simulink model "system_simulation"  (Simulink 8.9)
settings: Solver=ode4  StartTime=0.0  StopTime=300  FixedStep=0.01  RelTol=1e-3  EnableMultiTasking=on
values from neighbouring files (symbols this model uses):
  alpha_0 = 10*pi/180    (= 0.174532925199)    [para_initial.m]
  attitude_angle_0 = [5*pi/180;3*pi/180;-5*pi/180]    [para_initial.m]
  beta_0 = -10*pi/180    (= -0.174532925199)    [para_initial.m]
  omega_0 = 0.00075563    [para_initial.m]
  u_0 = [0;0;0;0;0;0;0;0]    [para_initial.m]
settings Model: Creator=Administrator  LastModifiedBy=yyywxk
settings DataIOCC: SignalLoggingSaveFormat=Dataset
settings DebuggingCC: SolverPrmCheckMsg=warning  MultiTaskDSMMsg=warning  MultiTaskCondExecSysMsg=none
settings GRTTargetCC: CombineOutputUpdateFcns=on  GRTInterface=off

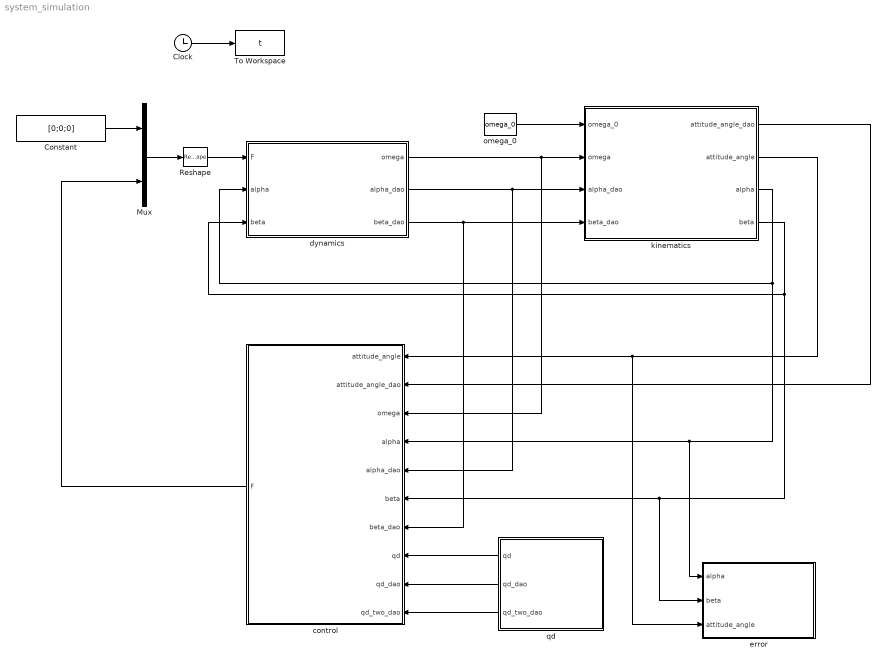
== system system_simulation ==
  Clock : Clock
  Constant : Constant  Value=[0;0;0]
  Mux : Mux  Inputs=2
  Reshape : Reshape
  To Workspace : ToWorkspace  VariableName=t  SampleTime=-1
  control : Subsystem
  dynamics : Subsystem
  error : Subsystem
  kinematics : Subsystem
  omega_0 : Constant  Value=omega_0
  qd : Subsystem
  wires:
  Clock/1 -> To Workspace/1
  dynamics/2(alpha_dao) -> control/5(alpha_dao), kinematics/3(alpha_dao)
  dynamics/1(omega) -> control/3(omega), kinematics/2(omega)
  omega_0/1 -> kinematics/1(omega_0)
  kinematics/3(alpha) -> dynamics/2(alpha), error/1(alpha), control/4(alpha)
  kinematics/2(attitude_angle) -> error/3(attitude_angle), control/1(attitude_angle)
  kinematics/1(attitude_angle_dao) -> control/2(attitude_angle_dao)
  Mux/1 -> Reshape/1
  Constant/1 -> Mux/1
  control/1(F) -> Mux/2
  Reshape/1 -> dynamics/1(F)
  dynamics/3(beta_dao) -> control/7(beta_dao), kinematics/4(beta_dao)
  qd/2(qd_dao) -> control/9(qd_dao)
  qd/1(qd) -> control/8(qd)
  qd/3(qd_two_dao) -> control/10(qd_two_dao)
  kinematics/4(beta) -> dynamics/3(beta), error/2(beta), control/6(beta)

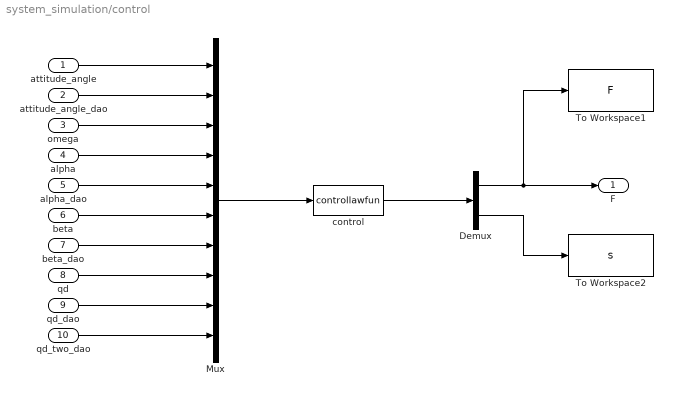
== system system_simulation/control ==
  attitude_angle : Inport
  attitude_angle_dao : Inport  Port=2
  omega : Inport  Port=3
  alpha : Inport  Port=4
  alpha_dao : Inport  Port=5
  beta : Inport  Port=6
  beta_dao : Inport  Port=7
  qd : Inport  Port=8
  qd_dao : Inport  Port=9
  qd_two_dao : Inport  Port=10
  Demux : Demux  Outputs=2
  Mux : Mux  Inputs=10
  To Workspace1 : ToWorkspace  VariableName=F  SampleTime=-1
  To Workspace2 : ToWorkspace  VariableName=s  SampleTime=-1
  control : MATLABFcn  MATLABFcn=controllawfun  OutputDimensions=10
  F : Outport
  wires:
  Mux/1 -> control/1
  attitude_angle/1 -> Mux/1
  attitude_angle_dao/1 -> Mux/2
  omega/1 -> Mux/3
  alpha/1 -> Mux/4
  alpha_dao/1 -> Mux/5
  qd/1 -> Mux/8
  qd_dao/1 -> Mux/9
  qd_two_dao/1 -> Mux/10
  control/1 -> Demux/1
  Demux/1 -> F/1, To Workspace1/1
  Demux/2 -> To Workspace2/1
  beta/1 -> Mux/6
  beta_dao/1 -> Mux/7

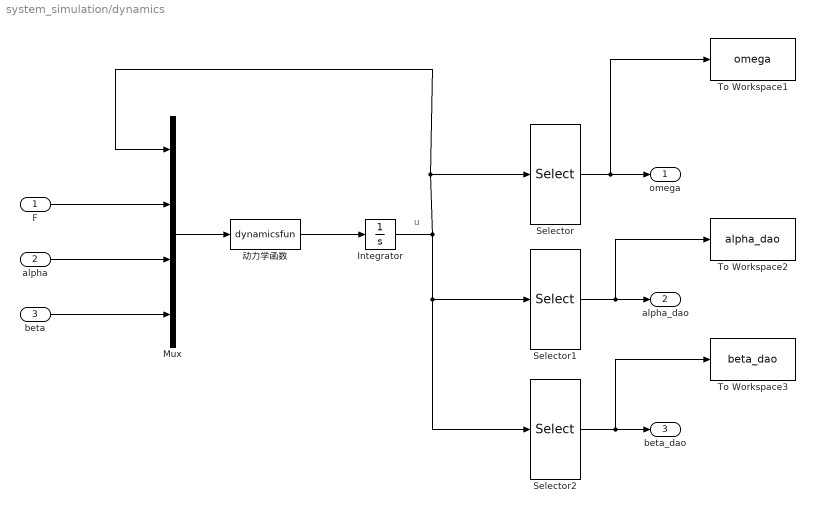
== system system_simulation/dynamics ==
  note: u
  F : Inport
  alpha : Inport  Port=2
  beta : Inport  Port=3
  Integrator : Integrator  InitialCondition=u_0
  Mux : Mux
  Selector : Selector  InputPortWidth=8  IndexOptions=Index vector (dialog)  Indices=[4 5 6]  OutputSizes=1
  Selector1 : Selector  InputPortWidth=8  IndexOptions=Index vector (dialog)  Indices=[7]  OutputSizes=1
  Selector2 : Selector  InputPortWidth=8  IndexOptions=Index vector (dialog)  Indices=[8]  OutputSizes=1
  To Workspace1 : ToWorkspace  VariableName=omega  SampleTime=-1
  To Workspace2 : ToWorkspace  VariableName=alpha_dao  SampleTime=-1
  To Workspace3 : ToWorkspace  VariableName=beta_dao  SampleTime=-1
  动力学函数 : MATLABFcn  MATLABFcn=dynamicsfun  OutputDimensions=8
  omega : Outport
  alpha_dao : Outport  Port=2
  beta_dao : Outport  Port=3
  wires:
  Mux/1 -> 动力学函数/1
  F/1 -> Mux/2
  alpha/1 -> Mux/3
  动力学函数/1 -> Integrator/1
  Integrator/1 -> Selector2/1, Selector1/1, Mux/1, Selector/1
  Selector/1 -> omega/1, To Workspace1/1
  Selector1/1 -> alpha_dao/1, To Workspace2/1
  Selector2/1 -> To Workspace3/1, beta_dao/1
  beta/1 -> Mux/4

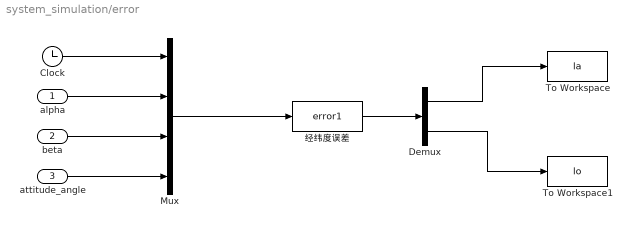
== system system_simulation/error ==
  alpha : Inport
  beta : Inport  Port=2
  attitude_angle : Inport  Port=3
  Clock : Clock
  Demux : Demux  Outputs=2
  Mux : Mux
  To Workspace : ToWorkspace  VariableName=la  SampleTime=-1
  To Workspace1 : ToWorkspace  VariableName=lo  SampleTime=-1
  经纬度误差 : MATLABFcn  MATLABFcn=error1  OutputDimensions=2
  wires:
  Clock/1 -> Mux/1
  Mux/1 -> 经纬度误差/1
  经纬度误差/1 -> Demux/1
  Demux/1 -> To Workspace/1
  Demux/2 -> To Workspace1/1
  alpha/1 -> Mux/2
  beta/1 -> Mux/3
  attitude_angle/1 -> Mux/4

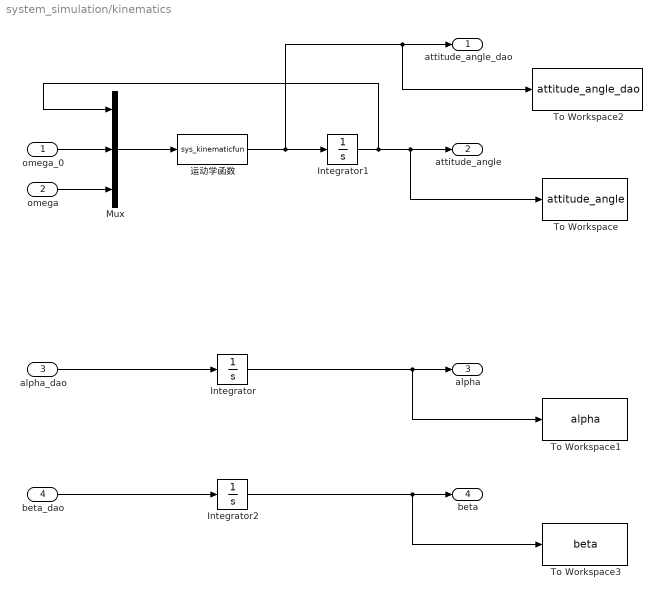
== system system_simulation/kinematics ==
  omega_0 : Inport
  omega : Inport  Port=2
  alpha_dao : Inport  Port=3
  beta_dao : Inport  Port=4
  Integrator : Integrator  InitialCondition=alpha_0
  Integrator1 : Integrator  InitialCondition=attitude_angle_0
  Integrator2 : Integrator  InitialCondition=beta_0
  Mux : Mux  Inputs=3
  To Workspace : ToWorkspace  VariableName=attitude_angle  SampleTime=-1
  To Workspace1 : ToWorkspace  VariableName=alpha  SampleTime=-1
  To Workspace2 : ToWorkspace  VariableName=attitude_angle_dao  SampleTime=-1
  To Workspace3 : ToWorkspace  VariableName=beta  SampleTime=-1
  运动学函数 : MATLABFcn  MATLABFcn=sys_kinematicfun  OutputDimensions=3
  attitude_angle_dao : Outport
  attitude_angle : Outport  Port=2
  alpha : Outport  Port=3
  beta : Outport  Port=4
  wires:
  Integrator/1 -> alpha/1, To Workspace1/1
  Integrator1/1 -> To Workspace/1, attitude_angle/1, Mux/1
  omega_0/1 -> Mux/2
  alpha_dao/1 -> Integrator/1
  omega/1 -> Mux/3
  Integrator2/1 -> beta/1, To Workspace3/1
  beta_dao/1 -> Integrator2/1
  Mux/1 -> 运动学函数/1
  运动学函数/1 -> To Workspace2/1, attitude_angle_dao/1, Integrator1/1

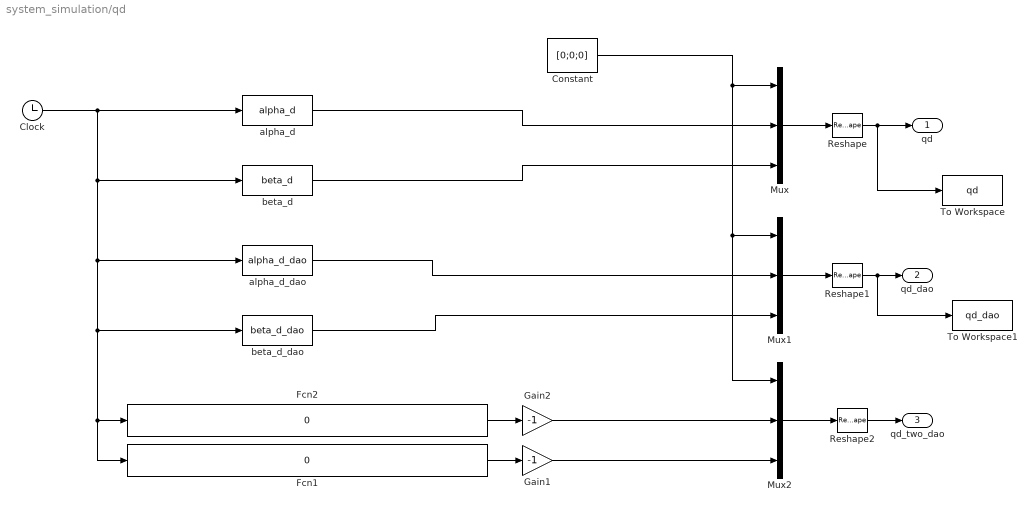
== system system_simulation/qd ==
  Clock : Clock
  Constant : Constant  Value=[0;0;0]
  Fcn1 : Fcn  Expr=0
  Fcn2 : Fcn  Expr=0
  Gain1 : Gain  Gain=-1
  Gain2 : Gain  Gain=-1
  Mux : Mux  Inputs=3
  Mux1 : Mux  Inputs=3
  Mux2 : Mux  Inputs=3
  Reshape : Reshape
  Reshape1 : Reshape
  Reshape2 : Reshape
  To Workspace : ToWorkspace  VariableName=qd  SampleTime=-1
  To Workspace1 : ToWorkspace  VariableName=qd_dao  SampleTime=-1
  alpha_d : MATLABFcn  MATLABFcn=alpha_d
  alpha_d_dao : MATLABFcn  MATLABFcn=alpha_d_dao
  "beta_d " : MATLABFcn  MATLABFcn=beta_d
  beta_d_dao : MATLABFcn  MATLABFcn=beta_d_dao
  qd : Outport
  qd_dao : Outport  Port=2
  qd_two_dao : Outport  Port=3
  wires:
  Constant/1 -> Mux/1, Mux1/1, Mux2/1
  Mux/1 -> Reshape/1
  Mux1/1 -> Reshape1/1
  Mux2/1 -> Reshape2/1
  Clock/1 -> "beta_d "/1, alpha_d_dao/1, beta_d_dao/1, Fcn2/1, Fcn1/1, alpha_d/1
  Fcn1/1 -> Gain1/1
  Reshape/1 -> qd/1, To Workspace/1
  Reshape1/1 -> To Workspace1/1, qd_dao/1
  Reshape2/1 -> qd_two_dao/1
  Fcn2/1 -> Gain2/1
  Gain2/1 -> Mux2/2
  Gain1/1 -> Mux2/3
  alpha_d/1 -> Mux/2
  "beta_d "/1 -> Mux/3
  alpha_d_dao/1 -> Mux1/2
  beta_d_dao/1 -> Mux1/3
